simulink library "PC_Simulator_Lib"  (Simulink 8.2)
settings: Solver=ode45  StartTime=0.0  StopTime=10.0  RelTol=1e-3
values from neighbouring files (symbols this model uses):
  data = [r1 r2 r3 r4 L1 L2 L3 L4]    [strasse_Bedatung_HNI_ITI.m]
  distSameLane = 60    [InitialisationsEnv.m]
  eng_speed = [0 60 120 180 240 300 360 420 480 540 600 660 ... (101 elements, 1x101)]    [engine_table.mat]    (also in motor_parameter_calc.m = omega)
  Heading_init = 0    [Start.m]
  inertiaLateral = 25*(radiusWheel)^2    (= 4.129024)    [Start.m]
  laneWidth = 3.6    [InitialisationsEnv.m]    (also in strasse_Bedatung_HNI_ITI.m)
  omega_engine = [0.000000 150.000000 500.000000 1000.000000 1500.000000 2000.000000 2500.000000 3000.000000 3500.000000 4000.000000 4500.000000 5000.000000 5500.000000 6000.000000]    [friction_tables.m]
  omega_max = 6000    [engine_table.mat]    (also in motor_parameter_calc.m)
  omega_wheel = [0 20 40 60 80 100 122 143.7 164]    [friction_tables.m]
  para_Fellow_8_Points = ADAS.Fellow_8_Points    [ADAS_parameters.m]
  position_start_x = [x1 x2 x3 x4 x5 x6 x7]    [strasse_Bedatung_HNI_ITI.m]
  position_start_y = [y1 y2 y3 y4 y5 y6 y7]    [strasse_Bedatung_HNI_ITI.m]
  rad3rdLine = 57.2    [InitialisationsEnv.m]    (also in strasse_Bedatung_HNI_ITI.m)
  radiusWheel = 16*2.54/100    (= 0.4064)    [Start.m]
  s_values = [S1 S2 S3 S4 S5 S6 S7]    [strasse_Bedatung_HNI_ITI.m]
  segmentLimits = [segment1EndThirdLine                   segment2EndThirdLine                   segment3EndThirdLine                   segment4EndThirdLine                   segment5EndThirdLine                   segment6EndThirdLine                   segment7EndThirdLine                   segment8EndThirdLine                   ]    [InitialisationsEnv.m]    (also in strasse_Bedatung_HNI_ITI.m)
  setPosT = [-1.8 -5.4 -1.8 -5.4 -1.8 -5.4 -1.8 -5.4 -1.8 -5.4]    [InitialisationsEnv.m]
  torque = [297.089227105 300.997600937 304.800343044 308.497453426 312.088932082 315.574779014 318.95499422 322.229577701 325.398529457 328.461849487 331.419537793 334.271594373 ... (101 elements, 1x101)]    [engine_table.mat]    (also in motor_parameter_calc.m = g)
  Torque_lost = [0.000000 -8.777780 -15.000000 -26.800000 -29.600000 -32.700000 -35.900000 -39.300000 -42.800000 -46.500000 -50.300000 -54.300000 -58.500000 -62.800000 ]*0.6    [friction_tables.m]
  Torque_lost_wheel = [0.8 0.8 0.75 0.7 0.4 0.3 0.2 0.07 0.07]*0.2    [friction_tables.m]
  X_init = 0    [Start.m]
  Y_init = 1.8    [Start.m]
  Z_init = 0    [Start.m]
undefined symbols (not defined in the file or in its folder): Acc_Pedal, ADAS, Brake_Pedal, Joystick, Newton, Para, Raphson, Standard_Devices, Steering_Wheel_Angle, UDP_Protocol
libraries: simulink x43, rtwinlib x7, dspnetwork x2, simulink_extras x1, vrlib x1
(part 10 of 13)

== system PC_Simulator_Lib/ADAS/Execution_ADAS/Longitudinal_Controller/Acceleration_Control/PI_Controller_plus_antiwindup_For_Trottel1 ==
  a_desired[m|s2] : Inport
  a_acctual[m|s2] : Inport  Port=2
  Difference_on_sides_Saturation : Inport  Port=3
  Brake_control_is_inactive[bool] : Inport  Port=4
  Gas_Pedal_Inverse_Motor[norm] : Inport  Port=5
  Abs : Abs
  Add : Sum
  Compare To Zero : simulink/Logic and Bit Operations/Compare To Zero  relop=>  OutDataTypeStr=uint8
  Compare To Zero1 : simulink/Logic and Bit Operations/Compare To Zero  relop=>  OutDataTypeStr=uint8
  Compare To Zero2 : simulink/Logic and Bit Operations/Compare To Zero  relop=~=  OutDataTypeStr=uint8
  Constant : Constant  Value=0
  Data Type Conversion : DataTypeConversion
  Data Type Conversion1 : DataTypeConversion
  Integrator : Integrator
  Ki : Gain  Gain=ADAS.Acceleration_Control.Throttel_PI.Ki
  Kp : Gain  Gain=ADAS.Acceleration_Control.Throttel_PI.Kp
  Logical Operator : Logic  AllPortsSameDT=off  OutDataTypeStr=boolean
  Product : Product  RndMeth=Zero
  Product1 : Product  Inputs=3
  Product2 : Product  Inputs=3
  Subtract1 : Sum  Inputs=+-
  Switch : Switch  Criteria=u2 > Threshold
  Gas_Pedal_Zusatz[norm] : Outport
  wires:
  Data Type Conversion1/1 -> Product2/3, Product1/3
  Compare To Zero2/1 -> Data Type Conversion1/1
  Gas_Pedal_Inverse_Motor[norm]/1 -> Compare To Zero2/1
  Data Type Conversion/1 -> Product1/2, Product2/2
  Product2/1 -> Gas_Pedal_Zusatz[norm]/1
  Logical Operator/1 -> Switch/2
  Add/1 -> Product2/1, Product/1
  Switch/1 -> Ki/1
  Brake_control_is_inactive[bool]/1 -> Data Type Conversion/1
  Subtract1/1 -> Product1/1
  Compare To Zero1/1 -> Logical Operator/1
  Product/1 -> Compare To Zero1/1
  Difference_on_sides_Saturation/1 -> Abs/1
  Compare To Zero/1 -> Logical Operator/2
  Abs/1 -> Compare To Zero/1
  Kp/1 -> Add/1
  Integrator/1 -> Add/2
  Ki/1 -> Integrator/1
  Product1/1 -> Kp/1, Switch/3, Product/2
  a_acctual[m|s2]/1 -> Subtract1/2
  a_desired[m|s2]/1 -> Subtract1/1
  Constant/1 -> Switch/1

== system PC_Simulator_Lib/ADAS/Execution_ADAS/Longitudinal_Controller/Acceleration_Control/Throttel_angle_calculation ==
  Torque_Engine_required[Nm] : Inport
  Omega_Engine[rad|s] : Inport  Port=2
  Divide : Product  Inputs=*/
  Engine_Map : Lookup_n-D  NumberOfTableDimensions=1  BreakpointsForDimension1=eng_speed  BeginIndexSearchUsingPreviousIndexResult=on  Table=torque  InputSameDT=on
  Gain1 : Gain  Gain=60/(2*pi)
  Saturation : Saturate  UpperLimit=1  LowerLimit=0
  Subtract : Sum  Inputs=+-
  frection : Lookup_n-D  NumberOfTableDimensions=1  BreakpointsForDimension1=omega_engine  BeginIndexSearchUsingPreviousIndexResult=on  Table=Torque_lost  InputSameDT=on
  throutle_angle[norm] : Outport
  wires:
  Gain1/1 -> Engine_Map/1, frection/1
  Omega_Engine[rad|s]/1 -> Gain1/1
  Engine_Map/1 -> Divide/2  "Torque_Engine_max[Nm]"
  Divide/1 -> Saturation/1
  Torque_Engine_required[Nm]/1 -> Subtract/1
  Saturation/1 -> throutle_angle[norm]/1
  frection/1 -> Subtract/2
  Subtract/1 -> Divide/1

== system PC_Simulator_Lib/ADAS/Execution_ADAS/Longitudinal_Controller/Acceleration_Control/Tractive_Force_Required_determination ==
  a_desired[m|s2] : Inport
  Vx_CoG[m|s] : Inport  Port=2
  omega_4_Wheels[rad|s] : Inport  Port=3
  Road_inclination[rad] : Inport  Port=4
  1/Wheel_Radius : Gain  Gain=1/radiusWheel
  Add : Sum
  Add1 : Sum  Inputs=+++
  Add2 : Sum  Inputs=++++
  Bus Selector : BusSelector  OutputSignals=Omega_FL[rad|s],Omega_FR[rad|s],Omega_RL[rad|s],Omega_RR[rad|s]
  Force_of_Aerodynamics : Subsystem
  Friction_FL : Subsystem
  Friction_FR : Subsystem
  Friction_RL : Subsystem
  Friction_RR : Subsystem
  Trigonometric Function : Trigonometry
  acceleration_of_gravity : Gain  Gain=Para.VD.gravity.v
  mass_Vehicle : Gain  Gain=Para.VD.Mass.v
  mass_Vehicle1 : Gain  Gain=Para.VD.Mass.v
  F_tire_required[N] : Outport
  wires:
  a_desired[m|s2]/1 -> mass_Vehicle/1
  mass_Vehicle/1 -> Add/1
  Add/1 -> F_tire_required[N]/1
  Add1/1 -> Add/2  "F_Load[N]"
  Vx_CoG[m|s]/1 -> Force_of_Aerodynamics/1(Vx_CoG[m|s])
  Force_of_Aerodynamics/1(Force_of_aerodynamics_in_X) -> Add1/1
  Bus Selector/1 -> Friction_FL/1(omega_radPs)  "<Omega_FL[rad|s]>"
  Bus Selector/2 -> Friction_FR/1(omega_radPs)  "<Omega_FR[rad|s]>"
  Bus Selector/3 -> Friction_RL/1(omega_radPs)  "<Omega_RL[rad|s]>"
  Bus Selector/4 -> Friction_RR/1(omega_radPs)  "<Omega_RR[rad|s]>"
  omega_4_Wheels[rad|s]/1 -> Bus Selector/1
  Friction_FL/1(Torque_friction) -> Add2/1
  Friction_FR/1(Torque_friction) -> Add2/2
  Friction_RL/1(Torque_friction) -> Add2/3
  Friction_RR/1(Torque_friction) -> Add2/4
  Add2/1 -> 1/Wheel_Radius/1
  1/Wheel_Radius/1 -> Add1/2
  Road_inclination[rad]/1 -> Trigonometric Function/1
  Trigonometric Function/1 -> mass_Vehicle1/1
  mass_Vehicle1/1 -> acceleration_of_gravity/1
  acceleration_of_gravity/1 -> Add1/3

== system PC_Simulator_Lib/ADAS/Sensors_ADAS/Front_Long_Range_Radar_Sensor/First_STage_Coordinate_Transformation/Radar_Triangles_Transformation_From_Local2Global ==
  Position_VUT_Vector[m] : Inport
  Oriantation_VUT_Vector[rad] : Inport  Port=2
  Apex : Constant  Value=LocPosTriang.Apex
  Bus Selector : BusSelector  OutputSignals=Roll_VUT[rad],Pitch_VUT[rad],Yaw_VUT[rad]
  Centeral_triangle_left : Constant  Value=LocPosTriang.Centeral_triangle_left
  Centeral_triangle_right : Constant  Value=LocPosTriang.Centeral_triangle_right
  Coord_Transformatin_Rotation : MATLAB Function  TreatAsAtomicUnit=on
  Coord_Transformatin_Rotation1 : MATLAB Function  TreatAsAtomicUnit=on
  Lower_triangle_left : Constant  Value=LocPosTriang.Lower_triangle_left
  Lower_triangle_right : Constant  Value=LocPosTriang.Lower_triangle_right
  Pitch_angle_offset : Subsystem
  Subsystem : Subsystem
  Subsystem1 : Subsystem
  Subsystem2 : Subsystem
  Subsystem3 : Subsystem
  Subsystem4 : Subsystem
  Subsystem5 : Subsystem
  Subsystem6 : Subsystem
  Subsystem7 : Subsystem
  Sum : Sum  Inputs=|++
  Upper_triangle_left : Constant  Value=LocPosTriang.Upper_triangle_left
  Upper_triangle_right : Constant  Value=LocPosTriang.Upper_triangle_right
  Apex_Position_Global_output[m] : Outport
  Apex_Position_Global[m] : Outport  Port=2
  Centeral_triangle_LeftPoint_Position_Global[m] : Outport  Port=3
  Centeral_triangle_RightPoint_Position_Global[m] : Outport  Port=4
  Upper_triangle_LeftPoint_Position_Global[m] : Outport  Port=5
  Upper_triangle_RightPoint_Position_Global[m] : Outport  Port=6
  Lower_triangle_LeftPoint_Position_Global[m] : Outport  Port=7
  Lower_triangle_RightPoint_Position_Global[m] : Outport  Port=8
  Round_done[bool] : Outport  Port=9
  wires:
  Coord_Transformatin_Rotation1/1(Trans_Local2Global) -> Subsystem7/1(Transformation_Local2Global)
  Subsystem7/1(Position_Global[m]) -> Apex_Position_Global_output[m]/1
  Pitch_angle_offset/2(Round_done[bool]) -> Round_done[bool]/1
  Pitch_angle_offset/1(Delta_pitch_angle[rad]) -> Sum/2
  Sum/1 -> Coord_Transformatin_Rotation/2(pitch)
  Oriantation_VUT_Vector[rad]/1 -> Bus Selector/1
  Bus Selector/2 -> Sum/1, Coord_Transformatin_Rotation1/2(pitch)  "<Pitch_VUT[rad]>"
  Bus Selector/1 -> Coord_Transformatin_Rotation/1(roll), Coord_Transformatin_Rotation1/1(roll)  "<Roll_VUT[rad]>"
  Bus Selector/3 -> Coord_Transformatin_Rotation/3(yaw), Coord_Transformatin_Rotation1/3(yaw)  "<Yaw_VUT[rad]>"
  Apex/1 -> Subsystem/3(Positon_Local[m]), Subsystem7/3(Positon_Local[m])
  Coord_Transformatin_Rotation/1(Trans_Local2Global) -> Subsystem1/1(Transformation_Local2Global), Subsystem2/1(Transformation_Local2Global), Subsystem3/1(Transformation_Local2Global), Subsystem4/1(Transformation_Local2Global), Subsystem6/1(Transformation_Local2Global), Subsystem5/1(Transformation_Local2Global), Subsystem/1(Transformation_Local2Global)
  Subsystem/1(Position_Global[m]) -> Apex_Position_Global[m]/1
  Subsystem1/1(Position_Global[m]) -> Centeral_triangle_LeftPoint_Position_Global[m]/1
  Subsystem2/1(Position_Global[m]) -> Centeral_triangle_RightPoint_Position_Global[m]/1
  Subsystem3/1(Position_Global[m]) -> Upper_triangle_LeftPoint_Position_Global[m]/1
  Subsystem4/1(Position_Global[m]) -> Upper_triangle_RightPoint_Position_Global[m]/1
  Subsystem5/1(Position_Global[m]) -> Lower_triangle_LeftPoint_Position_Global[m]/1
  Subsystem6/1(Position_Global[m]) -> Lower_triangle_RightPoint_Position_Global[m]/1
  Position_VUT_Vector[m]/1 -> Subsystem1/2(Position_of_Origine_Local_coord[m]), Subsystem2/2(Position_of_Origine_Local_coord[m]), Subsystem3/2(Position_of_Origine_Local_coord[m]), Subsystem4/2(Position_of_Origine_Local_coord[m]), Subsystem6/2(Position_of_Origine_Local_coord[m]), Subsystem5/2(Position_of_Origine_Local_coord[m]), Subsystem/2(Position_of_Origine_Local_coord[m]), Subsystem7/2(Position_of_Origine_Local_coord[m])
  Lower_triangle_right/1 -> Subsystem6/3(Positon_Local[m])
  Lower_triangle_left/1 -> Subsystem5/3(Positon_Local[m])
  Upper_triangle_right/1 -> Subsystem4/3(Positon_Local[m])
  Upper_triangle_left/1 -> Subsystem3/3(Positon_Local[m])
  Centeral_triangle_right/1 -> Subsystem2/3(Positon_Local[m])
  Centeral_triangle_left/1 -> Subsystem1/3(Positon_Local[m])

== system PC_Simulator_Lib/ADAS/Sensors_ADAS/Front_Long_Range_Radar_Sensor/First_STage_Coordinate_Transformation/Triangles_2_Fellows_Coord_Transformation_Plus_Sphere_Filtering ==
  Triangels_Points_Glob[m] : Inport
  Position_VUT_Vector[m] : Inport  Port=2
  Position_Fellows[m] : Inport  Port=3
  Oriantation_Fellows[rad] : Inport  Port=4
  MATLAB Function : MATLAB Function  TreatAsAtomicUnit=on
  Upper_Triangle_Vector[m] : Outport
  Centeral_Triangle_Vector[m] : Outport  Port=2
  Lower_Triangle_Vector[m] : Outport  Port=3
  Inside_Sphere_Vector[bool] : Outport  Port=4
  wires:
  Triangels_Points_Glob[m]/1 -> MATLAB Function/1(Triangles_Points_Glob)
  MATLAB Function/2(Central_Triangles) -> Centeral_Triangle_Vector[m]/1
  MATLAB Function/3(Lower_Triangles) -> Lower_Triangle_Vector[m]/1
  MATLAB Function/1(Upper_Triangles) -> Upper_Triangle_Vector[m]/1
  MATLAB Function/4(Inside_Sphere) -> Inside_Sphere_Vector[bool]/1
  Position_VUT_Vector[m]/1 -> MATLAB Function/4(Position_VUT)
  Position_Fellows[m]/1 -> MATLAB Function/2(Positon_Fellows)
  Oriantation_Fellows[rad]/1 -> MATLAB Function/3(Oriantation_Fellows)

== system PC_Simulator_Lib/ADAS/Sensors_ADAS/Front_Mid_Range_Radar_Sensor/First_STage_Coordinate_Transformation/Radar_Triangles_Transformation_From_Local2Global ==
  Position_VUT_Vector[m] : Inport
  Oriantation_VUT_Vector[rad] : Inport  Port=2
  Apex : Constant  Value=LocPosTriang.Apex
  Bus Selector : BusSelector  OutputSignals=Roll_VUT[rad],Pitch_VUT[rad],Yaw_VUT[rad]
  Centeral_triangle_left : Constant  Value=LocPosTriang.Centeral_triangle_left
  Centeral_triangle_right : Constant  Value=LocPosTriang.Centeral_triangle_right
  Coord_Transformatin_Rotation : MATLAB Function  TreatAsAtomicUnit=on
  Coord_Transformatin_Rotation1 : MATLAB Function  TreatAsAtomicUnit=on
  Lower_triangle_left : Constant  Value=LocPosTriang.Lower_triangle_left
  Lower_triangle_right : Constant  Value=LocPosTriang.Lower_triangle_right
  Pitch_angle_offset : Subsystem
  Subsystem : Subsystem
  Subsystem1 : Subsystem
  Subsystem2 : Subsystem
  Subsystem3 : Subsystem
  Subsystem4 : Subsystem
  Subsystem5 : Subsystem
  Subsystem6 : Subsystem
  Subsystem7 : Subsystem
  Sum : Sum  Inputs=|++
  Upper_triangle_left : Constant  Value=LocPosTriang.Upper_triangle_left
  Upper_triangle_right : Constant  Value=LocPosTriang.Upper_triangle_right
  Apex_Position_Global_output[m] : Outport
  Apex_Position_Global[m] : Outport  Port=2
  Centeral_triangle_LeftPoint_Position_Global[m] : Outport  Port=3
  Centeral_triangle_RightPoint_Position_Global[m] : Outport  Port=4
  Upper_triangle_LeftPoint_Position_Global[m] : Outport  Port=5
  Upper_triangle_RightPoint_Position_Global[m] : Outport  Port=6
  Lower_triangle_LeftPoint_Position_Global[m] : Outport  Port=7
  Lower_triangle_RightPoint_Position_Global[m] : Outport  Port=8
  Round_simulation_time[ms] : Outport  Port=9
  wires:
  Coord_Transformatin_Rotation1/1(Trans_Local2Global) -> Subsystem7/1(Transformation_Local2Global)
  Subsystem7/1(Position_Global[m]) -> Apex_Position_Global_output[m]/1
  Sum/1 -> Coord_Transformatin_Rotation/2(pitch)
  Pitch_angle_offset/2(Round_done[bool]) -> Round_simulation_time[ms]/1
  Pitch_angle_offset/1(Delta_pitch_angle[rad]) -> Sum/2
  Oriantation_VUT_Vector[rad]/1 -> Bus Selector/1
  Bus Selector/2 -> Sum/1, Coord_Transformatin_Rotation1/2(pitch)  "<Pitch_VUT[rad]>"
  Bus Selector/1 -> Coord_Transformatin_Rotation/1(roll), Coord_Transformatin_Rotation1/1(roll)  "<Roll_VUT[rad]>"
  Bus Selector/3 -> Coord_Transformatin_Rotation/3(yaw), Coord_Transformatin_Rotation1/3(yaw)  "<Yaw_VUT[rad]>"
  Apex/1 -> Subsystem/3(Positon_Local[m]), Subsystem7/3(Positon_Local[m])
  Coord_Transformatin_Rotation/1(Trans_Local2Global) -> Subsystem1/1(Transformation_Local2Global), Subsystem2/1(Transformation_Local2Global), Subsystem3/1(Transformation_Local2Global), Subsystem4/1(Transformation_Local2Global), Subsystem6/1(Transformation_Local2Global), Subsystem5/1(Transformation_Local2Global), Subsystem/1(Transformation_Local2Global)
  Subsystem/1(Position_Global[m]) -> Apex_Position_Global[m]/1
  Subsystem1/1(Position_Global[m]) -> Centeral_triangle_LeftPoint_Position_Global[m]/1
  Subsystem2/1(Position_Global[m]) -> Centeral_triangle_RightPoint_Position_Global[m]/1
  Subsystem3/1(Position_Global[m]) -> Upper_triangle_LeftPoint_Position_Global[m]/1
  Subsystem4/1(Position_Global[m]) -> Upper_triangle_RightPoint_Position_Global[m]/1
  Subsystem5/1(Position_Global[m]) -> Lower_triangle_LeftPoint_Position_Global[m]/1
  Subsystem6/1(Position_Global[m]) -> Lower_triangle_RightPoint_Position_Global[m]/1
  Position_VUT_Vector[m]/1 -> Subsystem1/2(Position_of_Origine_Local_coord[m]), Subsystem2/2(Position_of_Origine_Local_coord[m]), Subsystem3/2(Position_of_Origine_Local_coord[m]), Subsystem4/2(Position_of_Origine_Local_coord[m]), Subsystem6/2(Position_of_Origine_Local_coord[m]), Subsystem5/2(Position_of_Origine_Local_coord[m]), Subsystem/2(Position_of_Origine_Local_coord[m]), Subsystem7/2(Position_of_Origine_Local_coord[m])
  Lower_triangle_right/1 -> Subsystem6/3(Positon_Local[m])
  Lower_triangle_left/1 -> Subsystem5/3(Positon_Local[m])
  Upper_triangle_right/1 -> Subsystem4/3(Positon_Local[m])
  Upper_triangle_left/1 -> Subsystem3/3(Positon_Local[m])
  Centeral_triangle_right/1 -> Subsystem2/3(Positon_Local[m])
  Centeral_triangle_left/1 -> Subsystem1/3(Positon_Local[m])

== system PC_Simulator_Lib/ADAS/Sensors_ADAS/Front_Mid_Range_Radar_Sensor/First_STage_Coordinate_Transformation/Triangles_2_Fellows_Coord_Transformation_Plus_Sphere_Filtering ==
  Triangels_Points_Glob[m] : Inport
  Position_VUT_Vector[m] : Inport  Port=2
  Position_Fellows[m] : Inport  Port=3
  Oriantation_Fellows[rad] : Inport  Port=4
  MATLAB Function : MATLAB Function  TreatAsAtomicUnit=on
  Upper_Triangle_Vector[m] : Outport
  Centeral_Triangle_Vector[m] : Outport  Port=2
  Lower_Triangle_Vector[m] : Outport  Port=3
  Inside_Sphere_Vector[bool] : Outport  Port=4
  wires:
  Triangels_Points_Glob[m]/1 -> MATLAB Function/1(Triangles_Points_Glob)
  MATLAB Function/2(Central_Triangles) -> Centeral_Triangle_Vector[m]/1
  MATLAB Function/3(Lower_Triangles) -> Lower_Triangle_Vector[m]/1
  MATLAB Function/1(Upper_Triangles) -> Upper_Triangle_Vector[m]/1
  MATLAB Function/4(Inside_Sphere) -> Inside_Sphere_Vector[bool]/1
  Position_VUT_Vector[m]/1 -> MATLAB Function/4(Position_VUT)
  Position_Fellows[m]/1 -> MATLAB Function/2(Positon_Fellows)
  Oriantation_Fellows[rad]/1 -> MATLAB Function/3(Oriantation_Fellows)

== system PC_Simulator_Lib/ADAS/Sensors_ADAS/Input_Maping/Fellows/Subsystem1 ==
  Position_and_Oriantation_Fellows_Vector : Inport
  Bus Selector : BusSelector  OutputSignals=Vehicle_1_Vector.Vehicle_1_Gear_Angle[deg],Vehicle_2_Vector.Vehicle_2_Gear_Angle[deg],Vehicle_3_Vector.Vehicle_3_Gear_Angle[deg],Vehicle_4_Vector.Vehicle_4_Gear_Angle[deg],Vehicle_5_Vector.Vehicle_5_Gear_Angle[deg],Vehicle_6_Vector.Vehicle_6_Gear_Angle[deg],Vehicle_7_Vector.Vehicle_7_Gear_Angle[deg],Vehicle_8_Vector.Vehicle_8_Gear_Angle[deg],Vehicle_9_Vector.Vehicle_9_Gear_Angle[deg],Vehicle_10_Vector.Vehicle_10_Gear_Angle[deg]
  Constant : Constant  Value=0
  Gain{,1..9} (10 alike) : Gain  Gain=pi/180
  Mux : Mux  Inputs=30
  Oriantation_Fellows[m] : Outport
  wires:
  Position_and_Oriantation_Fellows_Vector/1 -> Bus Selector/1
  Mux/1 -> Oriantation_Fellows[m]/1
  Bus Selector/2 -> Gain1/1  "<Vehicle_2_Gear_Angle[deg]>"
  Bus Selector/1 -> Gain/1  "<Vehicle_1_Gear_Angle[deg]>"
  Bus Selector/3 -> Gain2/1  "<Vehicle_3_Gear_Angle[deg]>"
  Bus Selector/4 -> Gain3/1  "<Vehicle_4_Gear_Angle[deg]>"
  Bus Selector/5 -> Gain4/1  "<Vehicle_5_Gear_Angle[deg]>"
  Constant/1 -> Mux/16, Mux/29, Mux/28, Mux/26, Mux/25, Mux/23, Mux/22, Mux/20, Mux/19, Mux/17, Mux/14, Mux/13, Mux/11, Mux/10, Mux/8, Mux/7, Mux/5, Mux/4, Mux/2, Mux/1
  Bus Selector/6 -> Gain5/1  "<Vehicle_6_Gear_Angle[deg]>"
  Bus Selector/7 -> Gain6/1  "<Vehicle_7_Gear_Angle[deg]>"
  Bus Selector/8 -> Gain7/1  "<Vehicle_8_Gear_Angle[deg]>"
  Bus Selector/9 -> Gain8/1  "<Vehicle_9_Gear_Angle[deg]>"
  Bus Selector/10 -> Gain9/1  "<Vehicle_10_Gear_Angle[deg]>"
  Gain/1 -> Mux/3
  Gain1/1 -> Mux/6
  Gain9/1 -> Mux/30
  Gain8/1 -> Mux/27
  Gain7/1 -> Mux/24
  Gain6/1 -> Mux/21
  Gain5/1 -> Mux/18
  Gain4/1 -> Mux/15
  Gain3/1 -> Mux/12
  Gain2/1 -> Mux/9

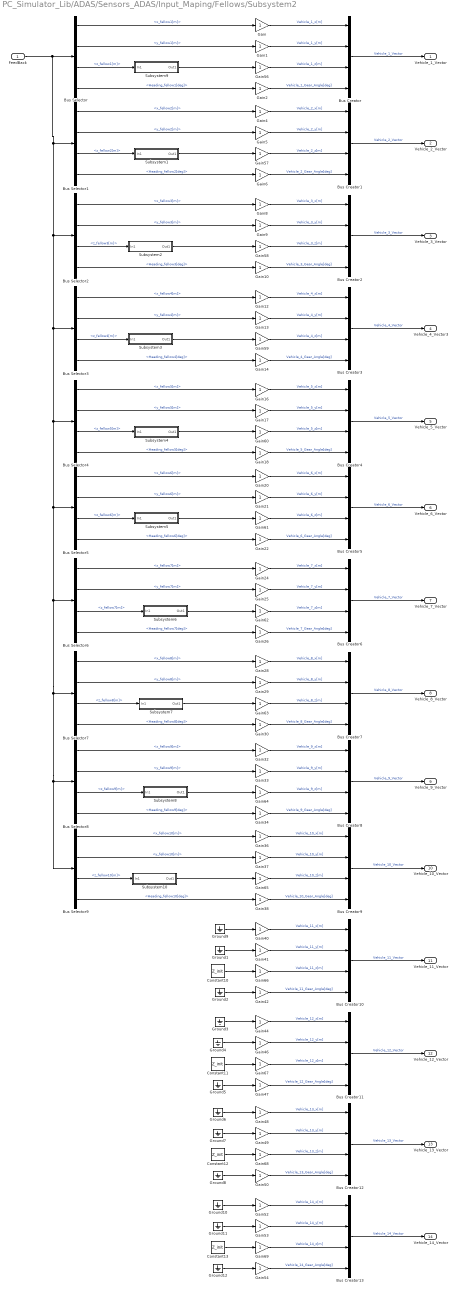
== system PC_Simulator_Lib/ADAS/Sensors_ADAS/Input_Maping/Fellows/Subsystem2 ==
  FeedBack : Inport
  Bus Creator{,1..13} (14 alike) : BusCreator
  Bus Selector : BusSelector  OutputSignals=Environment.fellow_car_1.x_fellow1[m],Environment.fellow_car_1.y_fellow1[m],Environment.fellow_car_1.z_fellow1[m],Environment.fellow_car_1.Heading_fellow1[deg]
  Bus Selector1 : BusSelector  OutputSignals=Environment.fellow_car_2.x_fellow2[m],Environment.fellow_car_2.y_fellow2[m],Environment.fellow_car_2.z_fellow2[m],Environment.fellow_car_2.Heading_fellow2[deg]
  Bus Selector2 : BusSelector  OutputSignals=Environment.fellow_car_3.x_fellow3[m],Environment.fellow_car_3.y_fellow3[m],Environment.fellow_car_3.z_fellow3[m],Environment.fellow_car_3.Heading_fellow3[deg]
  Bus Selector3 : BusSelector  OutputSignals=Environment.fellow_car_4.x_fellow4[m],Environment.fellow_car_4.y_fellow4[m],Environment.fellow_car_4.z_fellow4[m],Environment.fellow_car_4.Heading_fellow4[deg]
  Bus Selector4 : BusSelector  OutputSignals=Environment.fellow_car_5.x_fellow5[m],Environment.fellow_car_5.y_fellow5[m],Environment.fellow_car_5.z_fellow5[m],Environment.fellow_car_5.Heading_fellow5[deg]
  Bus Selector5 : BusSelector  OutputSignals=Environment.fellow_car_6.x_fellow6[m],Environment.fellow_car_6.y_fellow6[m],Environment.fellow_car_6.z_fellow6[m],Environment.fellow_car_6.Heading_fellow6[deg]
  Bus Selector6 : BusSelector  OutputSignals=Environment.fellow_car_7.x_fellow7[m],Environment.fellow_car_7.y_fellow7[m],Environment.fellow_car_7.z_fellow7[m],Environment.fellow_car_7.Heading_fellow7[deg]
  Bus Selector7 : BusSelector  OutputSignals=Environment.fellow_car_8.x_fellow8[m],Environment.fellow_car_8.y_fellow8[m],Environment.fellow_car_8.z_fellow8[m],Environment.fellow_car_8.Heading_fellow8[deg]
  Bus Selector8 : BusSelector  OutputSignals=Environment.fellow_car_9.x_fellow9[m],Environment.fellow_car_9.y_fellow9[m],Environment.fellow_car_9.z_fellow9[m],Environment.fellow_car_9.Heading_fellow9[deg]
  Bus Selector9 : BusSelector  OutputSignals=Environment.fellow_car_10.x_fellow10[m],Environment.fellow_car_10.y_fellow10[m],Environment.fellow_car_10.z_fellow10[m],Environment.fellow_car_10.Heading_fellow10[deg]
  Constant{10..13} (4 alike) : Constant  Value=Z_init
  Gain{,1..2,4..6,8..10,12..14,16..18,20..22,24..26,28..30,32..34,36..38,40..42,44,46..50,52..54,56..69} (56 alike) : Gain
  Ground{1..12} (12 alike) : Ground
  Subsystem1 : Subsystem
  Subsystem10 : Subsystem
  Subsystem2 : Subsystem
  Subsystem3 : Subsystem
  Subsystem4 : Subsystem
  Subsystem5 : Subsystem
  Subsystem6 : Subsystem
  Subsystem7 : Subsystem
  Subsystem8 : Subsystem
  Subsystem9 : Subsystem
  Vehicle_1_Vector : Outport
  Vehicle_2_Vector : Outport  Port=2
  Vehicle_3_Vector : Outport  Port=3
  Vehicle_4_Vector3 : Outport  Port=4
  Vehicle_5_Vector : Outport  Port=5
  Vehicle_6_Vector : Outport  Port=6
  Vehicle_7_Vector : Outport  Port=7
  Vehicle_8_Vector : Outport  Port=8
  Vehicle_9_Vector : Outport  Port=9
  Vehicle_10_Vector : Outport  Port=10
  Vehicle_11_Vector : Outport  Port=11
  Vehicle_12_Vector : Outport  Port=12
  Vehicle_13_Vector : Outport  Port=13
  Vehicle_14_Vector : Outport  Port=14
  wires:
  Bus Creator/1 -> Vehicle_1_Vector/1  "Vehicle_1_Vector"
  Bus Creator1/1 -> Vehicle_2_Vector/1  "Vehicle_2_Vector"
  Bus Creator2/1 -> Vehicle_3_Vector/1  "Vehicle_3_Vector"
  Bus Creator3/1 -> Vehicle_4_Vector3/1  "Vehicle_4_Vector"
  Bus Creator4/1 -> Vehicle_5_Vector/1  "Vehicle_5_Vector"
  Bus Creator5/1 -> Vehicle_6_Vector/1  "Vehicle_6_Vector"
  Bus Creator6/1 -> Vehicle_7_Vector/1  "Vehicle_7_Vector"
  Bus Creator7/1 -> Vehicle_8_Vector/1  "Vehicle_8_Vector"
  Bus Creator8/1 -> Vehicle_9_Vector/1  "Vehicle_9_Vector"
  Bus Creator9/1 -> Vehicle_10_Vector/1  "Vehicle_10_Vector"
  Bus Creator10/1 -> Vehicle_11_Vector/1  "Vehicle_11_Vector"
  Bus Creator11/1 -> Vehicle_12_Vector/1  "Vehicle_12_Vector"
  Bus Creator12/1 -> Vehicle_13_Vector/1  "Vehicle_13_Vector"
  Bus Creator13/1 -> Vehicle_14_Vector/1  "Vehicle_14_Vector"
  Gain/1 -> Bus Creator/1  "Vehicle_1_x[m]"
  Gain1/1 -> Bus Creator/2  "Vehicle_1_y[m]"
  Gain56/1 -> Bus Creator/3  "Vehicle_1_z[m]"
  Gain2/1 -> Bus Creator/4  "Vehicle_1_Gear_Angle[deg]"
  Gain4/1 -> Bus Creator1/1  "Vehicle_2_x[m]"
  Gain5/1 -> Bus Creator1/2  "Vehicle_2_y[m]"
  Gain57/1 -> Bus Creator1/3  "Vehicle_2_z[m]"
  Gain6/1 -> Bus Creator1/4  "Vehicle_2_Gear_Angle[deg]"
  Gain8/1 -> Bus Creator2/1  "Vehicle_3_x[m]"
  Gain9/1 -> Bus Creator2/2  "Vehicle_3_y[m]"
  Gain58/1 -> Bus Creator2/3  "Vehicle_3_z[m]"
  Gain10/1 -> Bus Creator2/4  "Vehicle_3_Gear_Angle[deg]"
  Gain12/1 -> Bus Creator3/1  "Vehicle_4_x[m]"
  Gain13/1 -> Bus Creator3/2  "Vehicle_4_y[m]"
  Gain59/1 -> Bus Creator3/3  "Vehicle_4_z[m]"
  Gain14/1 -> Bus Creator3/4  "Vehicle_4_Gear_Angle[deg]"
  Gain16/1 -> Bus Creator4/1  "Vehicle_5_x[m]"
  Gain17/1 -> Bus Creator4/2  "Vehicle_5_y[m]"
  Gain60/1 -> Bus Creator4/3  "Vehicle_5_z[m]"
  Gain18/1 -> Bus Creator4/4  "Vehicle_5_Gear_Angle[deg]"
  Gain20/1 -> Bus Creator5/1  "Vehicle_6_x[m]"
  Gain21/1 -> Bus Creator5/2  "Vehicle_6_y[m]"
  Gain61/1 -> Bus Creator5/3  "Vehicle_6_z[m]"
  Gain22/1 -> Bus Creator5/4  "Vehicle_6_Gear_Angle[deg]"
  Gain24/1 -> Bus Creator6/1  "Vehicle_7_x[m]"
  Gain25/1 -> Bus Creator6/2  "Vehicle_7_y[m]"
  Gain62/1 -> Bus Creator6/3  "Vehicle_7_z[m]"
  Gain26/1 -> Bus Creator6/4  "Vehicle_7_Gear_Angle[deg]"
  Gain28/1 -> Bus Creator7/1  "Vehicle_8_x[m]"
  Gain29/1 -> Bus Creator7/2  "Vehicle_8_y[m]"
  Gain63/1 -> Bus Creator7/3  "Vehicle_8_z[m]"
  Gain30/1 -> Bus Creator7/4  "Vehicle_8_Gear_Angle[deg]"
  Gain32/1 -> Bus Creator8/1  "Vehicle_9_x[m]"
  Gain33/1 -> Bus Creator8/2  "Vehicle_9_y[m]"
  Gain64/1 -> Bus Creator8/3  "Vehicle_9_z[m]"
  Gain34/1 -> Bus Creator8/4  "Vehicle_9_Gear_Angle[deg]"
  Gain36/1 -> Bus Creator9/1  "Vehicle_10_x[m]"
  Gain37/1 -> Bus Creator9/2  "Vehicle_10_y[m]"
  Gain65/1 -> Bus Creator9/3  "Vehicle_10_z[m]"
  Gain38/1 -> Bus Creator9/4  "Vehicle_10_Gear_Angle[deg]"
  Gain40/1 -> Bus Creator10/1  "Vehicle_11_x[m]"
  Gain41/1 -> Bus Creator10/2  "Vehicle_11_y[m]"
  Gain66/1 -> Bus Creator10/3  "Vehicle_11_z[m]"
  Gain42/1 -> Bus Creator10/4  "Vehicle_11_Gear_Angle[deg]"
  Gain44/1 -> Bus Creator11/1  "Vehicle_12_x[m]"
  Gain46/1 -> Bus Creator11/2  "Vehicle_12_y[m]"
  Gain67/1 -> Bus Creator11/3  "Vehicle_12_z[m]"
  Gain47/1 -> Bus Creator11/4  "Vehicle_12_Gear_Angle[deg]"
  Gain48/1 -> Bus Creator12/1  "Vehicle_13_x[m]"
  Gain49/1 -> Bus Creator12/2  "Vehicle_13_y[m]"
  Gain68/1 -> Bus Creator12/3  "Vehicle_13_z[m]"
  Gain50/1 -> Bus Creator12/4  "Vehicle_13_Gear_Angle[deg]"
  Gain52/1 -> Bus Creator13/1  "Vehicle_14_x[m]"
  Gain53/1 -> Bus Creator13/2  "Vehicle_14_y[m]"
  Gain69/1 -> Bus Creator13/3  "Vehicle_14_z[m]"
  Gain54/1 -> Bus Creator13/4  "Vehicle_14_Gear_Angle[deg]"
  Constant10/1 -> Gain66/1
  Constant11/1 -> Gain67/1
  Constant12/1 -> Gain68/1
  Constant13/1 -> Gain69/1
  FeedBack/1 -> Bus Selector9/1, Bus Selector8/1, Bus Selector7/1, Bus Selector6/1, Bus Selector5/1, Bus Selector4/1, Bus Selector3/1, Bus Selector2/1, Bus Selector1/1, Bus Selector/1
  Bus Selector/1 -> Gain/1  "<x_fellow1[m]>"
  Bus Selector/2 -> Gain1/1  "<y_fellow1[m]>"
  Bus Selector/3 -> Subsystem9/1(In1)  "<z_fellow1[m]>"
  Bus Selector/4 -> Gain2/1  "<Heading_fellow1[deg]>"
  Bus Selector1/1 -> Gain4/1  "<x_fellow2[m]>"
  Bus Selector1/2 -> Gain5/1  "<y_fellow2[m]>"
  Bus Selector1/3 -> Subsystem1/1(In1)  "<z_fellow2[m]>"
  Bus Selector1/4 -> Gain6/1  "<Heading_fellow2[deg]>"
  Bus Selector2/1 -> Gain8/1  "<x_fellow3[m]>"
  Bus Selector2/2 -> Gain9/1  "<y_fellow3[m]>"
  Bus Selector2/3 -> Subsystem2/1(In1)  "<z_fellow3[m]>"
  Bus Selector2/4 -> Gain10/1  "<Heading_fellow3[deg]>"
  Bus Selector3/1 -> Gain12/1  "<x_fellow4[m]>"
  Bus Selector3/2 -> Gain13/1  "<y_fellow4[m]>"
  Bus Selector3/3 -> Subsystem3/1(In1)  "<z_fellow4[m]>"
  Bus Selector3/4 -> Gain14/1  "<Heading_fellow4[deg]>"
  Bus Selector4/1 -> Gain16/1  "<x_fellow5[m]>"
  Bus Selector4/2 -> Gain17/1  "<y_fellow5[m]>"
  Bus Selector4/3 -> Subsystem4/1(In1)  "<z_fellow5[m]>"
  Bus Selector4/4 -> Gain18/1  "<Heading_fellow5[deg]>"
  Bus Selector5/1 -> Gain20/1  "<x_fellow6[m]>"
  Bus Selector5/2 -> Gain21/1  "<y_fellow6[m]>"
  Bus Selector5/3 -> Subsystem5/1(In1)  "<z_fellow6[m]>"
  Bus Selector5/4 -> Gain22/1  "<Heading_fellow6[deg]>"
  Bus Selector6/1 -> Gain24/1  "<x_fellow7[m]>"
  Bus Selector6/2 -> Gain25/1  "<y_fellow7[m]>"
  Bus Selector6/3 -> Subsystem6/1(In1)  "<z_fellow7[m]>"
  Bus Selector6/4 -> Gain26/1  "<Heading_fellow7[deg]>"
  Bus Selector7/1 -> Gain28/1  "<x_fellow8[m]>"
  Bus Selector7/2 -> Gain29/1  "<y_fellow8[m]>"
  Bus Selector7/3 -> Subsystem7/1(In1)  "<z_fellow8[m]>"
  Bus Selector7/4 -> Gain30/1  "<Heading_fellow8[deg]>"
  Bus Selector8/1 -> Gain32/1  "<x_fellow9[m]>"
  Bus Selector8/2 -> Gain33/1  "<y_fellow9[m]>"
  Bus Selector8/3 -> Subsystem8/1(In1)  "<z_fellow9[m]>"
  Bus Selector8/4 -> Gain34/1  "<Heading_fellow9[deg]>"
  Bus Selector9/1 -> Gain36/1  "<x_fellow10[m]>"
  Bus Selector9/2 -> Gain37/1  "<y_fellow10[m]>"
  Bus Selector9/3 -> Subsystem10/1(In1)  "<z_fellow10[m]>"
  Bus Selector9/4 -> Gain38/1  "<Heading_fellow10[deg]>"
  Ground9/1 -> Gain40/1
  Ground1/1 -> Gain41/1
  Ground2/1 -> Gain42/1
  Ground3/1 -> Gain44/1
  Ground4/1 -> Gain46/1
  Ground5/1 -> Gain47/1
  Ground6/1 -> Gain48/1
  Ground7/1 -> Gain49/1
  Ground8/1 -> Gain50/1
  Ground10/1 -> Gain52/1
  Ground11/1 -> Gain53/1
  Ground12/1 -> Gain54/1
  Subsystem9/1(Out1) -> Gain56/1
  Subsystem1/1(Out1) -> Gain57/1
  Subsystem2/1(Out1) -> Gain58/1
  Subsystem3/1(Out1) -> Gain59/1
  Subsystem4/1(Out1) -> Gain60/1
  Subsystem5/1(Out1) -> Gain61/1
  Subsystem6/1(Out1) -> Gain62/1
  Subsystem7/1(Out1) -> Gain63/1
  Subsystem8/1(Out1) -> Gain64/1
  Subsystem10/1(Out1) -> Gain65/1

== system PC_Simulator_Lib/ADAS/Sensors_ADAS/Input_Maping/Fellows/Subsystem3 ==
  Position_and_Oriantation_Fellows_Vector : Inport
  Bus Selector : BusSelector  OutputSignals=Vehicle_1_Vector.Vehicle_1_Gear_Angle[deg],Vehicle_2_Vector.Vehicle_2_Gear_Angle[deg],Vehicle_3_Vector.Vehicle_3_Gear_Angle[deg],Vehicle_4_Vector.Vehicle_4_Gear_Angle[deg],Vehicle_5_Vector.Vehicle_5_Gear_Angle[deg]
  Constant : Constant  Value=0
  Gain{,1..4} (5 alike) : Gain  Gain=pi/180
  Mux : Mux  Inputs=15
  Oriantation_Fellows[m] : Outport
  wires:
  Gain4/1 -> Mux/15
  Gain3/1 -> Mux/12
  Gain2/1 -> Mux/9
  Gain1/1 -> Mux/6
  Gain/1 -> Mux/3
  Bus Selector/5 -> Gain4/1  "<Vehicle_5_Gear_Angle[deg]>"
  Bus Selector/4 -> Gain3/1  "<Vehicle_4_Gear_Angle[deg]>"
  Bus Selector/3 -> Gain2/1  "<Vehicle_3_Gear_Angle[deg]>"
  Bus Selector/1 -> Gain/1  "<Vehicle_1_Gear_Angle[deg]>"
  Bus Selector/2 -> Gain1/1  "<Vehicle_2_Gear_Angle[deg]>"
  Constant/1 -> Mux/1, Mux/2, Mux/4, Mux/5, Mux/7, Mux/8, Mux/10, Mux/11, Mux/13, Mux/14
  Mux/1 -> Oriantation_Fellows[m]/1
  Position_and_Oriantation_Fellows_Vector/1 -> Bus Selector/1

== system PC_Simulator_Lib/ADAS/Sensors_ADAS/Input_Maping/Fellows/Subsystem4 ==
  Position_and_Oriantation_Fellows_Vector : Inport
  Bus Selector : BusSelector  OutputSignals=Vehicle_1_Vector.Vehicle_1_x[m],Vehicle_1_Vector.Vehicle_1_y[m],Vehicle_1_Vector.Vehicle_1_z[m],Vehicle_2_Vector.Vehicle_2_x[m],Vehicle_2_Vector.Vehicle_2_y[m],Vehicle_2_Vector.Vehicle_2_z[m],Vehicle_3_Vector.Vehicle_3_x[m],Vehicle_3_Vector.Vehicle_3_y[m],Vehicle_3_Vector.Vehicle_3_z[m],Vehicle_4_Vector.Vehicle_4_x[m],Vehicle_4_Vector.Vehicle_4_y[m],Vehicle_4_Vector.Vehicle_4_z[m],Vehicle_5_Vector.Vehicle_5_x[m],Vehicle_5_Vector.Vehicle_5_y[m],Vehicle_5_Vector.Vehicle_5_z[m]
  Mux : Mux  Inputs=15
  Position_Fellows[m] : Outport
  wires:
  Bus Selector/14 -> Mux/14  "<Vehicle_5_y[m]>"
  Bus Selector/10 -> Mux/10  "<Vehicle_4_x[m]>"
  Bus Selector/11 -> Mux/11  "<Vehicle_4_y[m]>"
  Bus Selector/13 -> Mux/13  "<Vehicle_5_x[m]>"
  Bus Selector/15 -> Mux/15  "<Vehicle_5_z[m]>"
  Bus Selector/12 -> Mux/12  "<Vehicle_4_z[m]>"
  Mux/1 -> Position_Fellows[m]/1
  Bus Selector/9 -> Mux/9  "<Vehicle_3_z[m]>"
  Bus Selector/8 -> Mux/8  "<Vehicle_3_y[m]>"
  Bus Selector/7 -> Mux/7  "<Vehicle_3_x[m]>"
  Bus Selector/6 -> Mux/6  "<Vehicle_2_z[m]>"
  Bus Selector/5 -> Mux/5  "<Vehicle_2_y[m]>"
  Bus Selector/4 -> Mux/4  "<Vehicle_2_x[m]>"
  Bus Selector/3 -> Mux/3  "<Vehicle_1_z[m]>"
  Bus Selector/2 -> Mux/2  "<Vehicle_1_y[m]>"
  Bus Selector/1 -> Mux/1  "<Vehicle_1_x[m]>"
  Position_and_Oriantation_Fellows_Vector/1 -> Bus Selector/1

== system PC_Simulator_Lib/ADAS/Sensors_ADAS/Input_Maping/Fellows/Subsystem5 ==
  Position_and_Oriantation_Fellows_Vector : Inport
  Bus Selector : BusSelector  OutputSignals=Vehicle_1_Vector.Vehicle_1_x[m],Vehicle_1_Vector.Vehicle_1_y[m],Vehicle_1_Vector.Vehicle_1_z[m],Vehicle_2_Vector.Vehicle_2_x[m],Vehicle_2_Vector.Vehicle_2_y[m],Vehicle_2_Vector.Vehicle_2_z[m],Vehicle_3_Vector.Vehicle_3_x[m],Vehicle_3_Vector.Vehicle_3_y[m],Vehicle_3_Vector.Vehicle_3_z[m],Vehicle_4_Vector.Vehicle_4_x[m],Vehicle_4_Vector.Vehicle_4_y[m],Vehicle_4_Vector.Vehicle_4_z[m],Vehicle_5_Vector.Vehicle_5_x[m],Vehicle_5_Vector.Vehicle_5_y[m],Vehicle_5_Vector.Vehicle_5_z[m],Vehicle_6_Vector.Vehicle_6_x[m],Vehicle_6_Vector.Vehicle_6_y[m],Vehicle_6_Vector.Vehicle_6_z[m],Vehicle_7_Vector.Vehicle_7_x[m],Vehicle_7_Vector.Vehicle_7_y[m],Vehicle_7_Vector.Vehicle_7_z[m],Vehicle_8_Vector.Vehicle_8_x[m],Vehicle_8_Vector.Vehicle_8_y[m],Vehicle_8_Vector.Vehicle_8_z[m],Vehicle_9_Vector.Vehicle_9_x[m],Vehicle_9_Vector.Vehicle_9_y[m],Vehicle_9_Vector.Vehicle_9_z[m],Vehicle_10_Vector.Vehicle_10_x[m],Vehicle_10_Vector.Vehicle_10_y[m],Vehicle_10_Vector.Vehicle_10_z[m]
  Mux : Mux  Inputs=30
  Position_Fellows[m] : Outport
  wires:
  Position_and_Oriantation_Fellows_Vector/1 -> Bus Selector/1
  Mux/1 -> Position_Fellows[m]/1
  Bus Selector/3 -> Mux/3  "<Vehicle_1_z[m]>"
  Bus Selector/7 -> Mux/7  "<Vehicle_3_x[m]>"
  Bus Selector/15 -> Mux/15  "<Vehicle_5_z[m]>"
  Bus Selector/1 -> Mux/1  "<Vehicle_1_x[m]>"
  Bus Selector/4 -> Mux/4  "<Vehicle_2_x[m]>"
  Bus Selector/6 -> Mux/6  "<Vehicle_2_z[m]>"
  Bus Selector/12 -> Mux/12  "<Vehicle_4_z[m]>"
  Bus Selector/5 -> Mux/5  "<Vehicle_2_y[m]>"
  Bus Selector/10 -> Mux/10  "<Vehicle_4_x[m]>"
  Bus Selector/9 -> Mux/9  "<Vehicle_3_z[m]>"
  Bus Selector/2 -> Mux/2  "<Vehicle_1_y[m]>"
  Bus Selector/13 -> Mux/13  "<Vehicle_5_x[m]>"
  Bus Selector/11 -> Mux/11  "<Vehicle_4_y[m]>"
  Bus Selector/8 -> Mux/8  "<Vehicle_3_y[m]>"
  Bus Selector/14 -> Mux/14  "<Vehicle_5_y[m]>"
  Bus Selector/29 -> Mux/29  "<Vehicle_10_y[m]>"
  Bus Selector/19 -> Mux/19  "<Vehicle_7_x[m]>"
  Bus Selector/18 -> Mux/18  "<Vehicle_6_z[m]>"
  Bus Selector/30 -> Mux/30  "<Vehicle_10_z[m]>"
  Bus Selector/21 -> Mux/21  "<Vehicle_7_z[m]>"
  Bus Selector/23 -> Mux/23  "<Vehicle_8_y[m]>"
  Bus Selector/28 -> Mux/28  "<Vehicle_10_x[m]>"
  Bus Selector/24 -> Mux/24  "<Vehicle_8_z[m]>"
  Bus Selector/20 -> Mux/20  "<Vehicle_7_y[m]>"
  Bus Selector/27 -> Mux/27  "<Vehicle_9_z[m]>"
  Bus Selector/26 -> Mux/26  "<Vehicle_9_y[m]>"
  Bus Selector/17 -> Mux/17  "<Vehicle_6_y[m]>"
  Bus Selector/25 -> Mux/25  "<Vehicle_9_x[m]>"
  Bus Selector/16 -> Mux/16  "<Vehicle_6_x[m]>"
  Bus Selector/22 -> Mux/22  "<Vehicle_8_x[m]>"

== system PC_Simulator_Lib/Drive_Train/4_Wheels_drive_train_and_Brake/FL/Alpha_Kappa_Selector2/Dynamik Anteil2 ==
  Fx : Inport
  Vx : Inport  Port=2
  omega : Inport  Port=3
  R : Inport  Port=4
  Abs : Abs
  Constant : Constant  Value=1000
  Constant1 : Constant  Value=1000
  Constant2 : Constant  Value=100
  Divide1 : Product  Inputs=*/
  Gain2 : Gain  Gain=-1
  Integrator : Integrator
  Integrator1 : Integrator
  Product : Product  RndMeth=Zero
  Product1 : Product  RndMeth=Zero
  Product2 : Product  RndMeth=Zero
  Product5 : Product  Inputs=*/  RndMeth=Zero
  Subsystem3 : Subsystem
  Sum : Sum  Inputs=|+-
  Sum1 : Sum  Inputs=|+-
  Sum2 : Sum  Inputs=|+--
  k : Outport
  wires:
  Constant2/1 -> Divide1/2
  R/1 -> Product/2
  Constant1/1 -> Product2/2  "<kcx>"
  Constant/1 -> Product1/2  "<dcx>"
  Fx/1 -> Sum2/1
  Abs/1 -> Subsystem3/1(In1)
  Divide1/1 -> Integrator1/1
  Sum2/1 -> Divide1/1
  Integrator1/1 -> Gain2/1, Sum1/1  "Vsxstern"
  Product1/1 -> Sum2/3
  Product2/1 -> Sum2/2
  Integrator/1 -> Product2/1
  Sum1/1 -> Integrator/1, Product1/1
  Sum/1 -> Sum1/2  "Vsx"
  Product/1 -> Sum/2
  Vx/1 -> Abs/1, Sum/1
  omega/1 -> Product/1
  Gain2/1 -> Product5/1
  Subsystem3/1(Out1) -> Product5/2
  Product5/1 -> k/1

== system PC_Simulator_Lib/Drive_Train/4_Wheels_drive_train_and_Brake/FL/Alpha_Kappa_Selector2/alpha_calc ==
  Vy : Inport
  Vx : Inport  Port=2
  Ground : Ground
  Slip_angle_Calculation_From_Vx_and_Vy1 : Subsystem
  Terminator : Terminator
  front : Subsystem
  alpha : Outport
  wires:
  Vx/1 -> Slip_angle_Calculation_From_Vx_and_Vy1/1(Vx_CoG[m|s]), front/2(Vx)
  Vy/1 -> Slip_angle_Calculation_From_Vx_and_Vy1/2(Vy_CoG[m|s]), front/1(Vy)
  front/1(alpha) -> Terminator/1
  Ground/1 -> front/3(steering_angle)
  Slip_angle_Calculation_From_Vx_and_Vy1/1(Slip_Angle[deg]) -> alpha/1

== system PC_Simulator_Lib/Drive_Train/4_Wheels_drive_train_and_Brake/FL/Wheel dynamics/Friction ==
  omega_radPs : Inport
  Lookup Table : Lookup_n-D  NumberOfTableDimensions=1  BreakpointsForDimension1=omega_wheel  BeginIndexSearchUsingPreviousIndexResult=on  Table=Torque_lost_wheel  InputSameDT=on
  Product : Product  RndMeth=Zero
  Torque_friction : Outport
  wires:
  omega_radPs/1 -> Product/2, Lookup Table/1
  Product/1 -> Torque_friction/1
  Lookup Table/1 -> Product/1

== system PC_Simulator_Lib/Drive_Train/4_Wheels_drive_train_and_Brake/FL/Wheel dynamics/Subsystem ==
  Torque_Brake_Nm : Inport
  Omega_rad/s : Inport  Port=2
  Compare To Constant : simulink/Logic and Bit Operations/Compare To Constant  relop=>=  const=0.1  OutDataTypeStr=uint8
  Compare To Constant1 : simulink/Logic and Bit Operations/Compare To Constant  relop=<=  const=-0.1  OutDataTypeStr=uint8
  Data Type Conversion : DataTypeConversion
  Logical Operator : Logic  Operator=OR  AllPortsSameDT=off  OutDataTypeStr=boolean
  Product : Product  Inputs=3  RndMeth=Zero
  Rate Limiter1 : RateLimiter  SampleTimeMode=inherited
  Sign : Signum
  Torque_Brake_act_Nm : Outport
  wires:
  Rate Limiter1/1 -> Product/3
  Compare To Constant1/1 -> Logical Operator/2
  Logical Operator/1 -> Data Type Conversion/1
  Data Type Conversion/1 -> Rate Limiter1/1
  Compare To Constant/1 -> Logical Operator/1
  Sign/1 -> Product/2
  Product/1 -> Torque_Brake_act_Nm/1
  Omega_rad/s/1 -> Sign/1, Compare To Constant/1, Compare To Constant1/1
  Torque_Brake_Nm/1 -> Product/1

== system PC_Simulator_Lib/Drive_Train/4_Wheels_drive_train_and_Brake/FR/Alpha_Kappa_Selector2/Dynamik Anteil2 ==
  Fx : Inport
  Vx : Inport  Port=2
  omega : Inport  Port=3
  R : Inport  Port=4
  Abs : Abs
  Constant : Constant  Value=1000
  Constant1 : Constant  Value=1000
  Constant2 : Constant  Value=100
  Divide1 : Product  Inputs=*/
  Gain2 : Gain  Gain=-1
  Integrator : Integrator
  Integrator1 : Integrator
  Product : Product  RndMeth=Zero
  Product1 : Product  RndMeth=Zero
  Product2 : Product  RndMeth=Zero
  Product5 : Product  Inputs=*/  RndMeth=Zero
  Subsystem3 : Subsystem
  Sum : Sum  Inputs=|+-
  Sum1 : Sum  Inputs=|+-
  Sum2 : Sum  Inputs=|+--
  k : Outport
  wires:
  Constant2/1 -> Divide1/2
  R/1 -> Product/2
  Constant1/1 -> Product2/2  "<kcx>"
  Constant/1 -> Product1/2  "<dcx>"
  Fx/1 -> Sum2/1
  Abs/1 -> Subsystem3/1(In1)
  Divide1/1 -> Integrator1/1
  Sum2/1 -> Divide1/1
  Integrator1/1 -> Gain2/1, Sum1/1  "Vsxstern"
  Product1/1 -> Sum2/3
  Product2/1 -> Sum2/2
  Integrator/1 -> Product2/1
  Sum1/1 -> Integrator/1, Product1/1
  Sum/1 -> Sum1/2  "Vsx"
  Product/1 -> Sum/2
  Vx/1 -> Abs/1, Sum/1
  omega/1 -> Product/1
  Gain2/1 -> Product5/1
  Subsystem3/1(Out1) -> Product5/2
  Product5/1 -> k/1

== system PC_Simulator_Lib/Drive_Train/4_Wheels_drive_train_and_Brake/FR/Alpha_Kappa_Selector2/alpha_calc ==
  Vy : Inport
  Vx : Inport  Port=2
  Ground : Ground
  Slip_angle_Calculation_From_Vx_and_Vy1 : Subsystem
  Terminator : Terminator
  front : Subsystem
  alpha : Outport
  wires:
  Vx/1 -> Slip_angle_Calculation_From_Vx_and_Vy1/1(Vx_CoG[m|s]), front/2(Vx)
  Vy/1 -> Slip_angle_Calculation_From_Vx_and_Vy1/2(Vy_CoG[m|s]), front/1(Vy)
  front/1(alpha) -> Terminator/1
  Ground/1 -> front/3(steering_angle)
  Slip_angle_Calculation_From_Vx_and_Vy1/1(Slip_Angle[deg]) -> alpha/1

== system PC_Simulator_Lib/Drive_Train/4_Wheels_drive_train_and_Brake/FR/Wheel dynamics/Friction ==
  omega_radPs : Inport
  Lookup Table : Lookup_n-D  NumberOfTableDimensions=1  BreakpointsForDimension1=omega_wheel  BeginIndexSearchUsingPreviousIndexResult=on  Table=Torque_lost_wheel  InputSameDT=on
  Product : Product  RndMeth=Zero
  Torque_friction : Outport
  wires:
  omega_radPs/1 -> Product/2, Lookup Table/1
  Product/1 -> Torque_friction/1
  Lookup Table/1 -> Product/1

== system PC_Simulator_Lib/Drive_Train/4_Wheels_drive_train_and_Brake/FR/Wheel dynamics/Subsystem ==
  Torque_Brake_Nm : Inport
  Omega_rad/s : Inport  Port=2
  Compare To Constant : simulink/Logic and Bit Operations/Compare To Constant  relop=>=  const=0.1  OutDataTypeStr=uint8
  Compare To Constant1 : simulink/Logic and Bit Operations/Compare To Constant  relop=<=  const=-0.1  OutDataTypeStr=uint8
  Data Type Conversion : DataTypeConversion
  Logical Operator : Logic  Operator=OR  AllPortsSameDT=off  OutDataTypeStr=boolean
  Product : Product  Inputs=3  RndMeth=Zero
  Rate Limiter1 : RateLimiter  SampleTimeMode=inherited
  Sign : Signum
  Torque_Brake_act_Nm : Outport
  wires:
  Rate Limiter1/1 -> Product/3
  Compare To Constant1/1 -> Logical Operator/2
  Logical Operator/1 -> Data Type Conversion/1
  Data Type Conversion/1 -> Rate Limiter1/1
  Compare To Constant/1 -> Logical Operator/1
  Sign/1 -> Product/2
  Product/1 -> Torque_Brake_act_Nm/1
  Omega_rad/s/1 -> Sign/1, Compare To Constant/1, Compare To Constant1/1
  Torque_Brake_Nm/1 -> Product/1

== system PC_Simulator_Lib/Drive_Train/4_Wheels_drive_train_and_Brake/RL/Alpha_Kappa_Selector2/Dynamik Anteil2 ==
  Fx : Inport
  Vx : Inport  Port=2
  omega : Inport  Port=3
  R : Inport  Port=4
  Abs : Abs
  Constant : Constant  Value=1000
  Constant1 : Constant  Value=1000
  Constant2 : Constant  Value=100
  Divide1 : Product  Inputs=*/
  Gain2 : Gain  Gain=-1
  Integrator : Integrator
  Integrator1 : Integrator
  Product : Product  RndMeth=Zero
  Product1 : Product  RndMeth=Zero
  Product2 : Product  RndMeth=Zero
  Product5 : Product  Inputs=*/  RndMeth=Zero
  Subsystem3 : Subsystem
  Sum : Sum  Inputs=|+-
  Sum1 : Sum  Inputs=|+-
  Sum2 : Sum  Inputs=|+--
  k : Outport
  wires:
  Constant2/1 -> Divide1/2
  R/1 -> Product/2
  Constant1/1 -> Product2/2  "<kcx>"
  Constant/1 -> Product1/2  "<dcx>"
  Fx/1 -> Sum2/1
  Abs/1 -> Subsystem3/1(In1)
  Divide1/1 -> Integrator1/1
  Sum2/1 -> Divide1/1
  Integrator1/1 -> Gain2/1, Sum1/1  "Vsxstern"
  Product1/1 -> Sum2/3
  Product2/1 -> Sum2/2
  Integrator/1 -> Product2/1
  Sum1/1 -> Integrator/1, Product1/1
  Sum/1 -> Sum1/2  "Vsx"
  Product/1 -> Sum/2
  Vx/1 -> Abs/1, Sum/1
  omega/1 -> Product/1
  Gain2/1 -> Product5/1
  Subsystem3/1(Out1) -> Product5/2
  Product5/1 -> k/1

== system PC_Simulator_Lib/Drive_Train/4_Wheels_drive_train_and_Brake/RL/Alpha_Kappa_Selector2/alpha_calc ==
  Vy : Inport
  Vx : Inport  Port=2
  Ground : Ground
  Slip_angle_Calculation_From_Vx_and_Vy1 : Subsystem
  Terminator : Terminator
  front : Subsystem
  alpha : Outport
  wires:
  Vx/1 -> Slip_angle_Calculation_From_Vx_and_Vy1/1(Vx_CoG[m|s]), front/2(Vx)
  Vy/1 -> Slip_angle_Calculation_From_Vx_and_Vy1/2(Vy_CoG[m|s]), front/1(Vy)
  front/1(alpha) -> Terminator/1
  Ground/1 -> front/3(steering_angle)
  Slip_angle_Calculation_From_Vx_and_Vy1/1(Slip_Angle[deg]) -> alpha/1

== system PC_Simulator_Lib/Drive_Train/4_Wheels_drive_train_and_Brake/RL/Wheel dynamics/Friction ==
  omega_radPs : Inport
  Lookup Table : Lookup_n-D  NumberOfTableDimensions=1  BreakpointsForDimension1=omega_wheel  BeginIndexSearchUsingPreviousIndexResult=on  Table=Torque_lost_wheel  InputSameDT=on
  Product : Product  RndMeth=Zero
  Torque_friction : Outport
  wires:
  omega_radPs/1 -> Product/2, Lookup Table/1
  Product/1 -> Torque_friction/1
  Lookup Table/1 -> Product/1

== system PC_Simulator_Lib/Drive_Train/4_Wheels_drive_train_and_Brake/RL/Wheel dynamics/Subsystem ==
  Torque_Brake_Nm : Inport
  Omega_rad/s : Inport  Port=2
  Compare To Constant : simulink/Logic and Bit Operations/Compare To Constant  relop=>=  const=0.1  OutDataTypeStr=uint8
  Compare To Constant1 : simulink/Logic and Bit Operations/Compare To Constant  relop=<=  const=-0.1  OutDataTypeStr=uint8
  Data Type Conversion : DataTypeConversion
  Logical Operator : Logic  Operator=OR  AllPortsSameDT=off  OutDataTypeStr=boolean
  Product : Product  Inputs=3  RndMeth=Zero
  Rate Limiter1 : RateLimiter  SampleTimeMode=inherited
  Sign : Signum
  Torque_Brake_act_Nm : Outport
  wires:
  Rate Limiter1/1 -> Product/3
  Compare To Constant1/1 -> Logical Operator/2
  Logical Operator/1 -> Data Type Conversion/1
  Data Type Conversion/1 -> Rate Limiter1/1
  Compare To Constant/1 -> Logical Operator/1
  Sign/1 -> Product/2
  Product/1 -> Torque_Brake_act_Nm/1
  Omega_rad/s/1 -> Sign/1, Compare To Constant/1, Compare To Constant1/1
  Torque_Brake_Nm/1 -> Product/1

== system PC_Simulator_Lib/Drive_Train/4_Wheels_drive_train_and_Brake/RR/Alpha_Kappa_Selector2/Dynamik Anteil2 ==
  Fx : Inport
  Vx : Inport  Port=2
  omega : Inport  Port=3
  R : Inport  Port=4
  Abs : Abs
  Constant : Constant  Value=1000
  Constant1 : Constant  Value=1000
  Constant2 : Constant  Value=100
  Divide1 : Product  Inputs=*/
  Gain2 : Gain  Gain=-1
  Integrator : Integrator
  Integrator1 : Integrator
  Product : Product  RndMeth=Zero
  Product1 : Product  RndMeth=Zero
  Product2 : Product  RndMeth=Zero
  Product5 : Product  Inputs=*/  RndMeth=Zero
  Subsystem3 : Subsystem
  Sum : Sum  Inputs=|+-
  Sum1 : Sum  Inputs=|+-
  Sum2 : Sum  Inputs=|+--
  k : Outport
  wires:
  Constant2/1 -> Divide1/2
  R/1 -> Product/2
  Constant1/1 -> Product2/2  "<kcx>"
  Constant/1 -> Product1/2  "<dcx>"
  Fx/1 -> Sum2/1
  Abs/1 -> Subsystem3/1(In1)
  Divide1/1 -> Integrator1/1
  Sum2/1 -> Divide1/1
  Integrator1/1 -> Gain2/1, Sum1/1  "Vsxstern"
  Product1/1 -> Sum2/3
  Product2/1 -> Sum2/2
  Integrator/1 -> Product2/1
  Sum1/1 -> Integrator/1, Product1/1
  Sum/1 -> Sum1/2  "Vsx"
  Product/1 -> Sum/2
  Vx/1 -> Abs/1, Sum/1
  omega/1 -> Product/1
  Gain2/1 -> Product5/1
  Subsystem3/1(Out1) -> Product5/2
  Product5/1 -> k/1

== system PC_Simulator_Lib/Drive_Train/4_Wheels_drive_train_and_Brake/RR/Alpha_Kappa_Selector2/alpha_calc ==
  Vy : Inport
  Vx : Inport  Port=2
  Ground : Ground
  Slip_angle_Calculation_From_Vx_and_Vy1 : Subsystem
  Terminator : Terminator
  front : Subsystem
  alpha : Outport
  wires:
  Vx/1 -> Slip_angle_Calculation_From_Vx_and_Vy1/1(Vx_CoG[m|s]), front/2(Vx)
  Vy/1 -> Slip_angle_Calculation_From_Vx_and_Vy1/2(Vy_CoG[m|s]), front/1(Vy)
  front/1(alpha) -> Terminator/1
  Ground/1 -> front/3(steering_angle)
  Slip_angle_Calculation_From_Vx_and_Vy1/1(Slip_Angle[deg]) -> alpha/1

== system PC_Simulator_Lib/Drive_Train/4_Wheels_drive_train_and_Brake/RR/Wheel dynamics/Friction ==
  omega_radPs : Inport
  Lookup Table : Lookup_n-D  NumberOfTableDimensions=1  BreakpointsForDimension1=omega_wheel  BeginIndexSearchUsingPreviousIndexResult=on  Table=Torque_lost_wheel  InputSameDT=on
  Product : Product  RndMeth=Zero
  Torque_friction : Outport
  wires:
  omega_radPs/1 -> Product/2, Lookup Table/1
  Product/1 -> Torque_friction/1
  Lookup Table/1 -> Product/1

== system PC_Simulator_Lib/Drive_Train/4_Wheels_drive_train_and_Brake/RR/Wheel dynamics/Subsystem ==
  Torque_Brake_Nm : Inport
  Omega_rad/s : Inport  Port=2
  Compare To Constant : simulink/Logic and Bit Operations/Compare To Constant  relop=>=  const=0.1  OutDataTypeStr=uint8
  Compare To Constant1 : simulink/Logic and Bit Operations/Compare To Constant  relop=<=  const=-0.1  OutDataTypeStr=uint8
  Data Type Conversion : DataTypeConversion
  Logical Operator : Logic  Operator=OR  AllPortsSameDT=off  OutDataTypeStr=boolean
  Product : Product  Inputs=3  RndMeth=Zero
  Rate Limiter1 : RateLimiter  SampleTimeMode=inherited
  Sign : Signum
  Torque_Brake_act_Nm : Outport
  wires:
  Rate Limiter1/1 -> Product/3
  Compare To Constant1/1 -> Logical Operator/2
  Logical Operator/1 -> Data Type Conversion/1
  Data Type Conversion/1 -> Rate Limiter1/1
  Compare To Constant/1 -> Logical Operator/1
  Sign/1 -> Product/2
  Product/1 -> Torque_Brake_act_Nm/1
  Omega_rad/s/1 -> Sign/1, Compare To Constant/1, Compare To Constant1/1
  Torque_Brake_Nm/1 -> Product/1

== system PC_Simulator_Lib/Environment/Environment_Model/Traffic_Vehicle_Model11/Vehicle_Model_t/Controller ==
  ResetSig[] : Inport
  t_diff : Inport  Port=2
  Integral Gain : Gain  Gain=0.01
  Integrator : Integrator  ExternalReset=rising
  Proportional Gain : Gain  Gain=1.5
  Sum1 : Sum
  v_ref : Outport
  wires:
  t_diff/1 -> Integral Gain/1, Proportional Gain/1
  Integral Gain/1 -> Integrator/1
  Integrator/1 -> Sum1/2
  Proportional Gain/1 -> Sum1/1
  Sum1/1 -> v_ref/1
  ResetSig[]/1 -> Integrator/2
